simulink model "modelWithSimscapeRobotAndEnvironmentDynamics"  (R2022a)
settings: Solver=daessc  StartTime=0.0  StopTime=16  MaxStep=0.1  RelTol=1e-2  AbsTol=1e-2
values from neighbouring files (symbols this model uses):
  configSequence = [-0.501061022402 -0.485319444061 0.447530394494 -0.0261030910079 -0.440724306093 0.594332377665 0.0114553342542 0 0 0.712315437264 -1.59156502907 -0.483414164072 ... (126 elements, 18x7)]    [abbExampleRSTVariables.mat]    (also in abbSavedConfigs.mat)
  dq0 = [0 0 0 0 0 0 0 0 0 0 0 0 ... (18 elements, 18x1)]    [abbExampleRSTVariables.mat]
  q0 = [-0.501061022402 -0.485319444061 0.447530394494 -0.0261030910079 -0.440724306093 0.594332377665 0.0114553342542 0 0 0.712315437264 -1.59156502907 -0.483414164072 ... (18 elements, 18x1)]    [abbExampleRSTVariables.mat]
  widgetDimensions = [0.02 0.02 0.07]    [abbExampleSMVariables.mat]
undefined symbols (not defined in the file or in its folder): CenterTable, Floor, LeftShelf, X, Y, Z
libraries: sm_lib x273, nesl_utility x75, robotmaniplib x3, robotcorelib x1
(part 1 of 8)
settings Model: PauseTimes=3.1  Creator=The MathWorks, Inc.  LastModifiedBy=The MathWorks, Inc.
settings SolverCC: AlgebraicLoopSolver=TrustRegion
settings DebuggingCC: UnconnectedInputMsg=warning  UnconnectedOutputMsg=warning  UnconnectedLineMsg=warning  SFMachineParentedDataDiag=warning

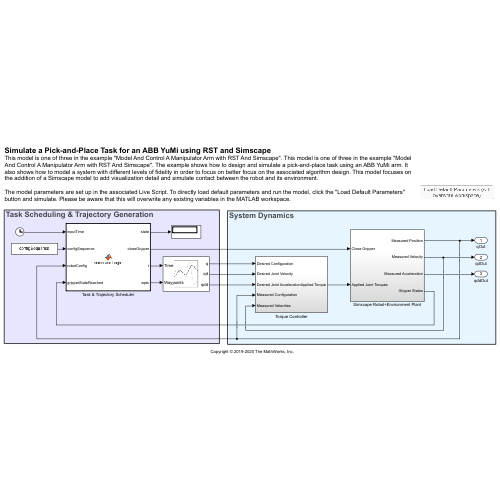
[thumbnail: Simulink's stored preview of the top-level diagram]
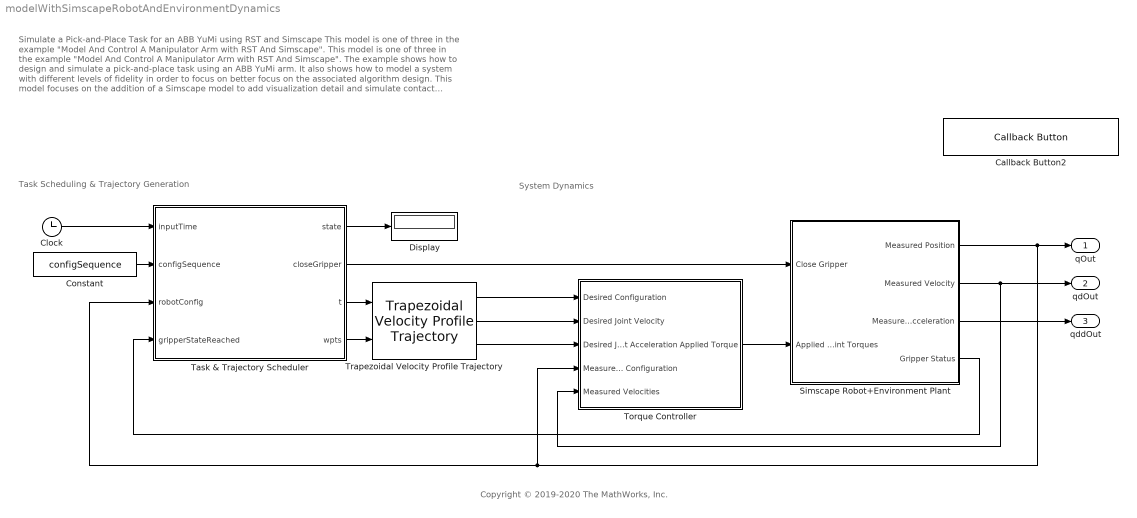
== system modelWithSimscapeRobotAndEnvironmentDynamics ==
  note: Copyright © 2019-2020 The MathWorks, Inc.
  note: Task Scheduling & Trajectory Generation
  note: System Dynamics
  note: Simulate a Pick-and-Place Task for an ABB YuMi using RST and Simscape
      | This model is one of three in the example "Model And Control A Manipulator Arm with RST And Simscape". This model is one of three in the example "Model And Control A Manipulator Arm with RST And Simscape". The example shows how to design and simulate a pick-and-place task using an ABB YuMi arm. It also shows how to model a system with different levels of fidelity in order to focus on better focus on the associated algorithm design. This model focuses on the addition of a Simscape model to add visualization detail and simulate contact between the robot and its environment.
      |
      | The model parameters are set up in the associated Live Script. To directly load default parameters and run the model, click the "Load Default Parameters" button and simulate. Please be aware that this will overwrite any existing variables in the MATLAB workspace.
  Callback Button2 : CallbackButton  ButtonText=Load Default Parameters (will overwrite workspace)
      settings: ClickFcn=|
      | robot = loadrobot('abbYumi', 'Gravity', [0 0 -9.81]);
      | load abbExampleRSTVariables.mat;
      | load abbExampleSMVariables.mat;
  Clock : Clock
  Constant : Constant  Value=configSequence
  Display : Display
  Simscape Robot+Environment Plant : Subsystem
  Task & Trajectory Scheduler : MATLAB Function  TreatAsAtomicUnit=on
  Torque Controller : Subsystem
  Trapezoidal Velocity Profile Trajectory : robotcorelib/Trapezoidal Velocity Profile Trajectory  WaypointSource=External  Waypoints=[ 0, -0.5, -1; 0, 0.5, 1 ]  NumParams=1  Parameter1=End Time  Parameter2=End Time  ParameterSource=Internal  PeakVelocity=[ 2; 2 ]  Acceleration=[ 1; 2 ]  EndTime=2  AccelTime=[ 1; 2 ]  SimulateUsing=Interpreted execution
      settings: SourceProductBaseCode=RO,NV,RR,UV
  qOut : Outport
  qdOut : Outport  Port=2
  qddOut : Outport  Port=3
  wires:
  Task & Trajectory Scheduler/1(state) -> Display/1
  Simscape Robot+Environment Plant/1(Measured Position) -> Torque Controller/4(Measured Configuration), Task & Trajectory Scheduler/3(robotConfig), qOut/1
  Simscape Robot+Environment Plant/2(Measured Velocity) -> Torque Controller/5(Measured Velocities), qdOut/1
  Simscape Robot+Environment Plant/3(Measured Acceleration) -> qddOut/1
  Simscape Robot+Environment Plant/4(Gripper Status) -> Task & Trajectory Scheduler/4(gripperStateReached)
  Clock/1 -> Task & Trajectory Scheduler/1(inputTime)
  Constant/1 -> Task & Trajectory Scheduler/2(configSequence)
  Task & Trajectory Scheduler/4(wpts) -> Trapezoidal Velocity Profile Trajectory/2
  Task & Trajectory Scheduler/3(t) -> Trapezoidal Velocity Profile Trajectory/1
  Trapezoidal Velocity Profile Trajectory/1 -> Torque Controller/1(Desired Configuration)
  Trapezoidal Velocity Profile Trajectory/2 -> Torque Controller/2(Desired Joint Velocity)
  Trapezoidal Velocity Profile Trajectory/3 -> Torque Controller/3(Desired Joint Acceleration)
  Torque Controller/1(Applied Torque) -> Simscape Robot+Environment Plant/2(Applied Joint Torques)
  Task & Trajectory Scheduler/2(closeGripper) -> Simscape Robot+Environment Plant/1(Close Gripper)

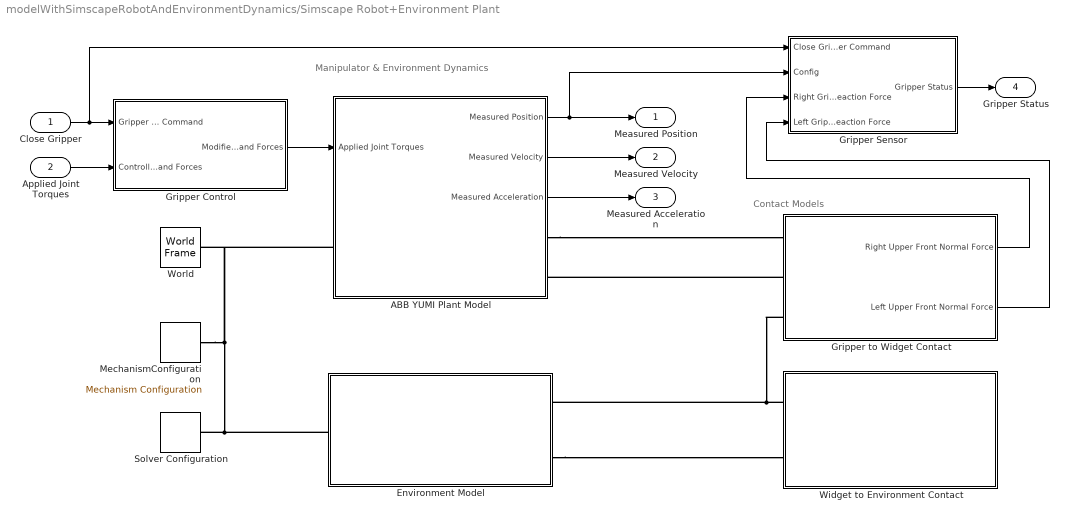
== system modelWithSimscapeRobotAndEnvironmentDynamics/Simscape Robot+Environment Plant ==
  note: Contact Models
  note: Manipulator & Environment Dynamics
  Close Gripper : Inport
  Applied Joint Torques : Inport  Port=2
  ABB YUMI Plant Model : Subsystem
  Environment Model : Subsystem
  Gripper Control : Subsystem
  Gripper Sensor : Subsystem
  Gripper to Widget Contact : Subsystem
  MechanismConfiguration : sm_lib/Utilities/Mechanism Configuration  UniformGravity=Constant  GravityVector=[0 0 -9.80665]  GravityUnits=m/s^2  LinearizationDelta=0.001  JointModeTransitionNonlinearIterations=2
  Solver Configuration : nesl_utility/Solver Configuration  PhysicalDomain=network_engine_domain  SubClassName=solver  LeftPortType=input  RightPortType=generic  Tones=[]  Harmonics=[]  SimulateNoise=off  Profile=off  UseLocalSampling=off  EnableSwitchedLinearOptims=on  FrequencyDomain=off  UseCCode=off  RelTol=0.001  AbsTol=1e-06  MinStep=1e-09  ToWorkspace=off  RevertToSquareIcSolve=off  NumHomotopyIterations=100  PhasorMode=off  PhasorModeNumHarmonics=1  IndexReductionMethod=DerivativeReplacement  DoDC=off  ResidualTolerance=1e-09  UseLocalSolver=off  LocalSolverChoice=NE_BACKWARD_EULER_ADVANCER  LocalSolverSampleTime=0.001  DoFixedCost=off  MaxNonlinIter=3  MaxModeIter=2  ComputeImpulses=off  ImpulseIterations=2  LinearAlgebra=auto  LinearAlgebraNumThread=0  EquationFormulation=NE_TIME_EF  DelaysMemoryBudget=1024  AutomaticFiltering=on  FilteringTimeConstant=0.001  PartitionStorageMethod=AS_NEEDED  PartitionMemoryBudget=1024  PartitionMethod=ROBUST
      settings: SourceProductBaseCode=SS,PW,VE
  Widget to Environment Contact : Subsystem
  World : sm_lib/Frames and Transforms/World Frame
  Measured Position : Outport
  Measured Velocity : Outport  Port=2
  Measured Acceleration : Outport  Port=3
  Gripper Status : Outport  Port=4
  wires:
  ABB YUMI Plant Model/1(Measured Position) -> Gripper Sensor/2(Config), Measured Position/1
  ABB YUMI Plant Model/2(Measured Velocity) -> Measured Velocity/1
  ABB YUMI Plant Model/3(Measured Acceleration) -> Measured Acceleration/1
  Gripper Control/1(Modified Joint Torques and Forces) -> ABB YUMI Plant Model/1(Applied Joint Torques)
  Applied Joint Torques/1 -> Gripper Control/2(Controller Joint Torques and Forces)
  Close Gripper/1 -> Gripper Sensor/1(Close Gripper Command), Gripper Control/1(Gripper Close Command)
  Gripper to Widget Contact/1(Right Upper Front Normal Force) -> Gripper Sensor/3(Right Gripper Reaction Force)
  Gripper to Widget Contact/2(Left Upper Front Normal Force) -> Gripper Sensor/4(Left Gripper Reaction Force)
  Gripper Sensor/1(Gripper Status) -> Gripper Status/1
  connections:
  MechanismConfiguration/RConn1 -- Solver Configuration/RConn1 -- Environment Model/LConn1 -- ABB YUMI Plant Model/LConn1 -- World/RConn1
  Gripper to Widget Contact/LConn3 -- Environment Model/RConn1 -- Widget to Environment Contact/LConn1
  Environment Model/RConn2 -- Widget to Environment Contact/LConn2
  ABB YUMI Plant Model/RConn1 -- Gripper to Widget Contact/LConn1
  Gripper to Widget Contact/LConn2 -- ABB YUMI Plant Model/RConn2

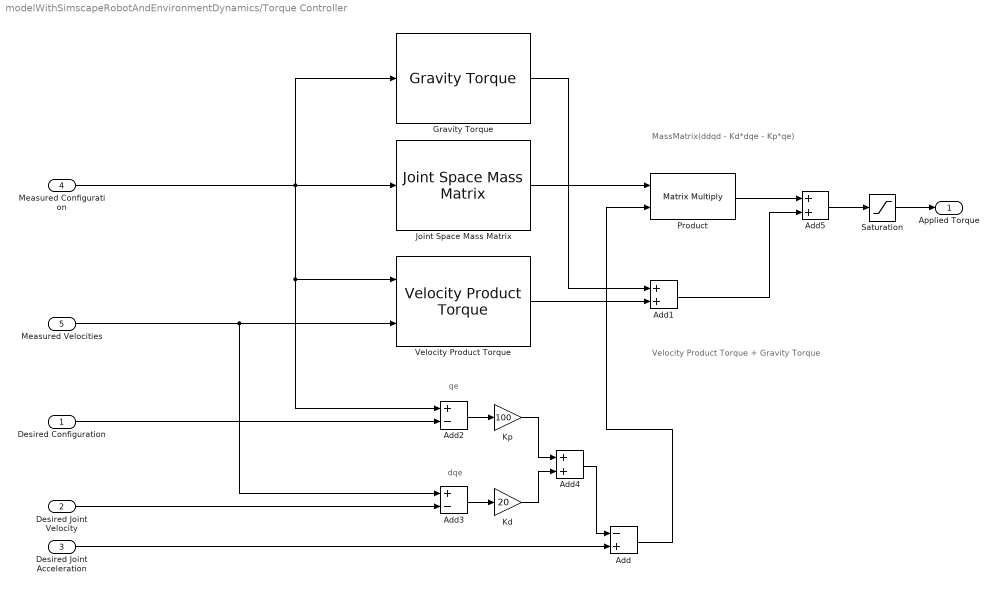
== system modelWithSimscapeRobotAndEnvironmentDynamics/Torque Controller ==
  note: qe
  note: dqe
  note: Velocity Product Torque + Gravity Torque
  note: MassMatrix(ddqd - Kd*dqe - Kp*qe)
  Desired Configuration : Inport
  Desired Joint Velocity : Inport  Port=2
  Desired Joint Acceleration : Inport  Port=3
  Measured Configuration : Inport  Port=4
  Measured Velocities : Inport  Port=5
  Add : Sum  Inputs=-+
  Add1 : Sum
  Add2 : Sum  Inputs=+-
  Add3 : Sum  Inputs=+-
  Add4 : Sum
  Add5 : Sum
  Gravity Torque : robotmaniplib/Gravity Torque  RigidBodyTree=robot  SimulateUsing=Interpreted execution
  Joint Space Mass Matrix : robotmaniplib/Joint Space Mass Matrix  RigidBodyTree=robot  SimulateUsing=Interpreted execution
  Kd : Gain  Gain=20
  Kp : Gain  Gain=100
  Product : Product  Multiplication=Matrix(*)
  Saturation : Saturate  UpperLimit=100  LowerLimit=-100
  Velocity Product Torque : robotmaniplib/Velocity Product Torque  RigidBodyTree=robot  SimulateUsing=Interpreted execution
      settings: SourceProductBaseCode=RO
  Applied Torque : Outport  VectorParamsAs1DForOutWhenUnconnected=off
  wires:
  Desired Joint Acceleration/1 -> Add/2
  Desired Joint Velocity/1 -> Add3/2
  Desired Configuration/1 -> Add2/2
  Joint Space Mass Matrix/1 -> Product/1
  Measured Configuration/1 -> Joint Space Mass Matrix/1, Gravity Torque/1, Velocity Product Torque/1, Add2/1
  Measured Velocities/1 -> Add3/1, Velocity Product Torque/2
  Add4/1 -> Add/1
  Add/1 -> Product/2
  Add2/1 -> Kp/1
  Add3/1 -> Kd/1
  Kp/1 -> Add4/1
  Kd/1 -> Add4/2
  Add5/1 -> Saturation/1
  Product/1 -> Add5/1
  Add1/1 -> Add5/2
  Gravity Torque/1 -> Add1/1
  Velocity Product Torque/1 -> Add1/2
  Saturation/1 -> Applied Torque/1
